simulink model "SIMULINK_LAB1"  (R2023a)
settings: Solver=VariableStepAuto  StartTime=0.0  StopTime=10.0  RelTol=1e-3
settings Model: Creator=mazen  LastModifiedBy=mazen

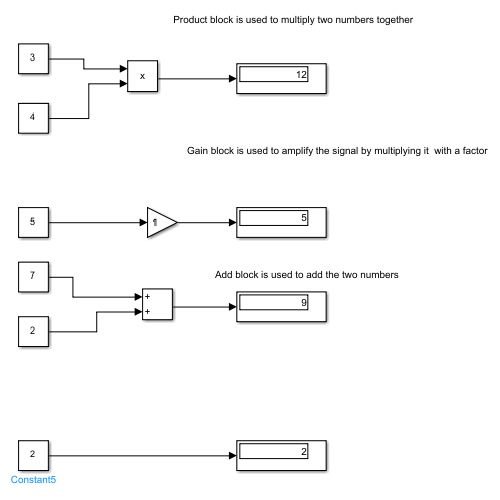
[thumbnail: Simulink's stored preview of the top-level diagram]
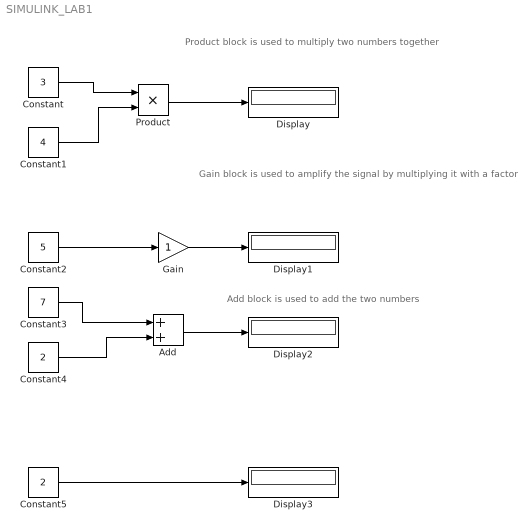
== system SIMULINK_LAB1 ==
  note: Add block is used to add the two numbers
  note: Gain block is used to amplify the signal by multiplying it with a factor
  note: Product block is used to multiply two numbers together
  Add : Sum
  Constant : Constant  Value=3
  Constant1 : Constant  Value=4
  Constant2 : Constant  Value=5
  Constant3 : Constant  Value=7
  Constant4 : Constant  Value=2
  Constant5 : Constant  Value=2
  Display{,1..3} (4 alike) : Display
  Gain : Gain
  Product : Product
  wires:
  Constant/1 -> Product/1
  Constant1/1 -> Product/2
  Product/1 -> Display/1
  Constant2/1 -> Gain/1
  Gain/1 -> Display1/1
  Constant4/1 -> Add/2
  Constant3/1 -> Add/1
  Add/1 -> Display2/1
  Constant5/1 -> Display3/1
